simulink model "ControlBA"  (R2023b)
settings: Solver=VariableStepAuto  StartTime=0.0  StopTime=10.0  RelTol=1e-3
settings Model: Creator=USUARIO  LastModifiedBy=USUARIO

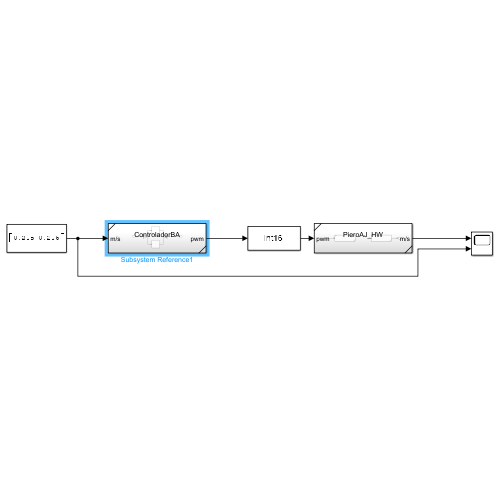
[thumbnail: Simulink's stored preview of the top-level diagram]
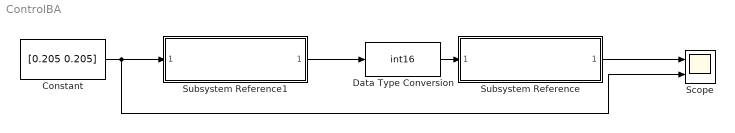
== system ControlBA ==
  Constant : Constant  Value=[0.205 0.205]
  Data Type Conversion : DataTypeConversion  OutDataTypeStr=int16  SaturateOnIntegerOverflow=off  RndMeth=Floor
  Scope : Scope  NumInputPorts=2
  Subsystem Reference : Subsystem  ReferencedSubsystem=PieroAJ_HW
  Subsystem Reference1 : Subsystem  ReferencedSubsystem=ControladorBA
  wires:
  Data Type Conversion/1 -> Subsystem Reference/1
  Subsystem Reference/1 -> Scope/1
  Constant/1 -> Subsystem Reference1/1, Scope/2
  Subsystem Reference1/1 -> Data Type Conversion/1
